simulink model "test_pi_flocking_xy_gazebo_2023a"  (R2023a)
settings: Solver=FixedStepAuto  StartTime=0.0  StopTime=inf  RelTol=1e-3
undefined symbols (not defined in the file or in its folder): angular, d_prime, DiscIntNeverNeededParam, epsilon, h, linear, R, vxobs, vyobs, vzobs, xobs, yobs, zobs
libraries: ros2lib x14, simulink x4, robotcorelib x4
(part 2 of 2)

== matlab function test_pi_flocking_xy_gazebo_2023a/Translational Control3/Flocking1/MATLAB Function4 ==
  data: xj input; yj input; zj input; vxj input; vyj input; vzj input; xk input; yk input; zk input; vxk input; vyk input; vzk input; xl input; yl input; zl input; vxl input; vyl input; vzl input; xobs parameter; yobs parameter; zobs parameter; phiBetaniknei output; R parameter; epsilon parameter; d_prime parameter; h parameter; vxobs parameter; vyobs parameter; vzobs parameter; bikve output
function [phiBetaniknei, bikve] = phiBetaFcn(xj, yj, zj, vxj, vyj, vzj, xk, yk, zk, vxk, vyk, vzk, xl, yl, zl, vxl, vyl, vzl, xobs, yobs, zobs, R, epsilon, d_prime, h, vxobs, vyobs, vzobs)
    
    dBeta = sigmaNormFun(d_prime, epsilon) ;
    
    Pj = [xj ; yj ; zj] ;
    Pk = [xk ; yk ; zk] ;
    Pl = [xl ; yl ; zl] ;
    Pc = [xobs ; yobs ; zobs] ;

    Vj = [vxj ; vyj ; vzj] ;
    Vk = [vxk ; vyk ; vzk] ;
    Vl = [vxl ; vyl ; vzl] ;
    Vc = [vxobs ; vyobs ; vzobs] ;

    % Compute closest point between the robot center and the obstacle
    % circumference (ossumming obstacles are circles)
    Pobsj = Pc + (Pj - Pc) * (R /norm(Pj - Pc)) ;
    Pobsk = Pc + (Pk - Pc) * (R /norm(Pk - Pc)) ;
    Pobsl = Pc + (Pl - Pc) * (R /norm(Pl - Pc)) ;
    %Pk = [xobs ; yobs] ;
    
    %%
    sigmaNormj = sigmaNormFun(Pobsj - Pj, epsilon) ;
    nij = gradSigmaFun(Pobsj - Pj, epsilon) ;
    
    sigmaNormk = sigmaNormFun(Pobsk - Pk, epsilon) ;
    nik = gradSigmaFun(Pobsk - Pk, epsilon) ;

    sigmaNorml = sigmaNormFun(Pobsl - Pl, epsilon) ;
    nil = gradSigmaFun(Pobsl - Pl, epsilon) ;

    %%
    sigma1j = sigma1Fun(sigmaNormj - dBeta) ;
    sigma1k = sigma1Fun(sigmaNormk - dBeta) ;
    sigma1l = sigma1Fun(sigmaNorml - dBeta) ;
            
    %%
    phiBetaj = bumpFcn(sigmaNormj/dBeta,h) * (sigma1j - 1) ;
    phiBetak = bumpFcn(sigmaNormk/dBeta,h) * (sigma1k - 1) ;
    phiBetal = bumpFcn(sigmaNorml/dBeta,h) * (sigma1l - 1) ;
            
    %% Position
    phiBetaniknei = phiBetaj.* nij + phiBetak.* nik + phiBetal.* nil;
    
    %% Velocity
    bikve = bumpFcn(sigmaNormj/dBeta,h).*(Vc + (Vj - Vc)) + bumpFcn(sigmaNormk/dBeta,h).*(Vc + (Vk - Vc)) + bumpFcn(sigmaNorml/dBeta,h).*(Vc + (Vl - Vc));
end

== matlab function test_pi_flocking_xy_gazebo_2023a/Translational Control4/Flocking1/MATLAB Function ==
  data: xi input; yi input; phiAlpha output; xj input; yj input; xk input; yk input; xl input; yl input; params input

function phiAlpha  = phiAlphaFcn(xi, yi, xj, yj, xk, yk, xl, yl, params)
    
    % Flocking parameters
    epsilon = params(1); a = params(2); b = params(3); c = params(4); d = params(5); h = params(6);

    e = abs(a - b) / sqrt(4*a*b) ;

    cAlpha = sigmaNormFun(c, epsilon) ;
    dAlpha = sigmaNormFun(d, epsilon) ;

    %%
    Pi = [xi;yi] ;
    Pj = [xj;yj] ;
    Pk = [xk;yk] ;
    Pl = [xl;yl] ;

    %%
    sigmaNormj = sigmaNormFun(Pj - Pi, epsilon) ;
    nij = gradSigmaFun(Pj - Pi, epsilon) ;
    
    sigmaNormk = sigmaNormFun(Pk - Pi, epsilon) ;
    nik = gradSigmaFun(Pk - Pi, epsilon) ;

    sigmaNorml = sigmaNormFun(Pl - Pi, epsilon) ;
    nil = gradSigmaFun(Pl - Pi, epsilon) ;

    %%
    sigma1j = sigma1Fun(sigmaNormj - dAlpha + e) ;
    sigma1k = sigma1Fun(sigmaNormk - dAlpha + e) ;
    sigma1l = sigma1Fun(sigmaNorml - dAlpha + e) ;
            
    %% Position
    phiAlphaj = 0.5 * bumpFcn(sigmaNormj/cAlpha,h) * ((a+b)*sigma1j + (a-b)) ;
    phiAlphanij = phiAlphaj.* nij ;
    
    phiAlphak = 0.5 * bumpFcn(sigmaNormk/cAlpha,h) * ((a+b)*sigma1k + (a-b)) ;
    phiAlphanik = phiAlphak.* nik ;

    phiAlphal = 0.5 * bumpFcn(sigmaNorml/cAlpha,h) * ((a+b)*sigma1l + (a-b)) ;
    phiAlphanil = phiAlphal.* nil ;

    phiAlpha = phiAlphanij + phiAlphanik + phiAlphanil;

    
end

== matlab function test_pi_flocking_xy_gazebo_2023a/Translational Control4/Flocking1/MATLAB Function1 ==
  data: phiAlpha input; phiAlpha_int input; ui_gamma input; yaw input; ieyaw input; Ui_pos output size=3; ui_yaw output; KP input; eyaw output

function [Ui_pos, ui_yaw, eyaw]  = ctrlLaw(phiAlpha, phiAlpha_int, ui_gamma, yaw, ieyaw, KP)  %, phiBetak, bikobs, phiBetanei, bikve
    
    % Control gains and parameters
    Kx = KP(1); Ky = KP(2); Kz = KP(3);
    Kix = KP(4); Kiy = KP(5); Kiz = KP(6);
    Kyaw = KP(7); Kdyaw = KP(8); Kiyaw = KP(9);
    
    hx_dot = Kx * phiAlpha(1,1) + Kix * phiAlpha_int(1,1) + ui_gamma(1,1);  %+ cBetax * (phiBetak(1,1) + phiBetanei(1,1)) + cdBetax * (bikobs(1,1) + bikve(1,1));
    hy_dot = Ky * phiAlpha(2,1) + Kiy * phiAlpha_int(2,1) + ui_gamma(2,1);  %+ cBetay * (phiBetak(2,1) + phiBetanei(2,1)) + cdBetay * (bikobs(2,1) + bikve(2,1));
    hz_dot = ui_gamma(3,1);  %+ cBetaz * (phiBetak(3,1) + phiBetanei(3,1)) + cdBetaz * (bikobs(3,1) + bikve(3,1));
    

    eyaw = 0 - yaw(1);
    deyaw = 0 - yaw(2);
    

    Ui_pos = [hx_dot; hy_dot; hz_dot] ;
    ui_yaw = Kyaw*eyaw + Kdyaw*deyaw + Kiyaw*ieyaw;

end

== matlab function test_pi_flocking_xy_gazebo_2023a/Translational Control1/Flocking1/MATLAB Function ==
  data: xi input; yi input; phiAlpha output; xj input; yj input; xk input; yk input; xl input; yl input; params input

function phiAlpha  = phiAlphaFcn(xi, yi, xj, yj, xk, yk, xl, yl, params)
    
    % Flocking parameters
    epsilon = params(1); a = params(2); b = params(3); c = params(4); d = params(5); h = params(6);

    e = abs(a - b) / sqrt(4*a*b) ;

    cAlpha = sigmaNormFun(c, epsilon) ;
    dAlpha = sigmaNormFun(d, epsilon) ;

    %%
    Pi = [xi;yi] ;
    Pj = [xj;yj] ;
    Pk = [xk;yk] ;
    Pl = [xl;yl] ;

    %%
    sigmaNormj = sigmaNormFun(Pj - Pi, epsilon) ;
    nij = gradSigmaFun(Pj - Pi, epsilon) ;
    
    sigmaNormk = sigmaNormFun(Pk - Pi, epsilon) ;
    nik = gradSigmaFun(Pk - Pi, epsilon) ;

    sigmaNorml = sigmaNormFun(Pl - Pi, epsilon) ;
    nil = gradSigmaFun(Pl - Pi, epsilon) ;

    %%
    sigma1j = sigma1Fun(sigmaNormj - dAlpha + e) ;
    sigma1k = sigma1Fun(sigmaNormk - dAlpha + e) ;
    sigma1l = sigma1Fun(sigmaNorml - dAlpha + e) ;
            
    %% Position
    phiAlphaj = 0.5 * bumpFcn(sigmaNormj/cAlpha,h) * ((a+b)*sigma1j + (a-b)) ;
    phiAlphanij = phiAlphaj.* nij ;
    
    phiAlphak = 0.5 * bumpFcn(sigmaNormk/cAlpha,h) * ((a+b)*sigma1k + (a-b)) ;
    phiAlphanik = phiAlphak.* nik ;

    phiAlphal = 0.5 * bumpFcn(sigmaNorml/cAlpha,h) * ((a+b)*sigma1l + (a-b)) ;
    phiAlphanil = phiAlphal.* nil ;

    phiAlpha = phiAlphanij + phiAlphanik + phiAlphanil;

    
end

== matlab function test_pi_flocking_xy_gazebo_2023a/Translational Control1/Flocking1/MATLAB Function1 ==
  data: phiAlpha input; phiAlpha_int input; ui_gamma input; yaw input; ieyaw input; Ui_pos output size=3; ui_yaw output; KP input; eyaw output

function [Ui_pos, ui_yaw, eyaw]  = ctrlLaw(phiAlpha, phiAlpha_int, ui_gamma, yaw, ieyaw, KP)  %, phiBetak, bikobs, phiBetanei, bikve
    
    % Control gains and parameters
    Kx = KP(1); Ky = KP(2); Kz = KP(3);
    Kix = KP(4); Kiy = KP(5); Kiz = KP(6);
    Kyaw = KP(7); Kdyaw = KP(8); Kiyaw = KP(9);
    
    hx_dot = Kx * phiAlpha(1,1) + Kix * phiAlpha_int(1,1) + ui_gamma(1,1);  %+ cBetax * (phiBetak(1,1) + phiBetanei(1,1)) + cdBetax * (bikobs(1,1) + bikve(1,1));
    hy_dot = Ky * phiAlpha(2,1) + Kiy * phiAlpha_int(2,1) + ui_gamma(2,1);  %+ cBetay * (phiBetak(2,1) + phiBetanei(2,1)) + cdBetay * (bikobs(2,1) + bikve(2,1));
    hz_dot = ui_gamma(3,1);  %+ cBetaz * (phiBetak(3,1) + phiBetanei(3,1)) + cdBetaz * (bikobs(3,1) + bikve(3,1));
    

    eyaw = 0 - yaw(1);
    deyaw = 0 - yaw(2);
    

    Ui_pos = [hx_dot; hy_dot; hz_dot] ;
    ui_yaw = Kyaw*eyaw + Kdyaw*deyaw + Kiyaw*ieyaw;

end

== matlab function test_pi_flocking_xy_gazebo_2023a/Translational Control1/Flocking1/MATLAB Function2 ==
  data: xi input; yi input; zi input; ui_gamma output; xr input; yr input; zr input; iep input size=3; ep output size=3; K_cts input

function [ui_gamma, ep] = naviFeedback(xi, yi, zi, xr, yr, zr, iep, K_cts)
    
    Kp = K_cts(1); Ki = K_cts(2);
    xmin = K_cts(3); xmax = K_cts(4);
       
    Pi = [xi ; yi ; zi] ;
    
    Pr = [xr ; yr ; zr] ;
    
    ep = Pi - Pr;
    
    ui_gamma = (-1).* satFcn(Kp.*(ep), xmin, xmax) + (-1).* satFcn(Ki.*(iep), xmin, xmax) ;
    
end

== matlab function test_pi_flocking_xy_gazebo_2023a/Translational Control1/Flocking1/MATLAB Function3 ==
  data: xi input; yi input; zi input; vxi input; vyi input; vzi input; xobs parameter; yobs parameter; zobs parameter; vxobs parameter; vyobs parameter; vzobs parameter; phiBetanik output; R parameter; epsilon parameter; d_prime parameter; h parameter; bikobs output
function [phiBetanik, bikobs] = phiBetaFcn(xi, yi, zi, vxi, vyi, vzi, xobs, yobs, zobs, vxobs, vyobs, vzobs, R, epsilon, d_prime, h)
    
    dBeta = sigmaNormFun(d_prime, epsilon) ;
    
    Pi = [xi ; yi ; zi] ;
    Pc = [xobs ; yobs ; zobs] ;
    
    Vi = [vxi ; vyi ; vzi] ;
    Vc = [vxobs ; vyobs ; vzobs] ;

    % Compute closest point between the robot center and the obstacle
    % circumference (ossumming obstacles are circles)
    Pk = Pc + (Pi - Pc) * (R /norm(Pi - Pc)) ;
    %Pk = [xobs ; yobs] ;
    
    sigmaNormk = sigmaNormFun(Pk - Pi, epsilon) ;
    nik = gradSigmaFun(Pk - Pi, epsilon) ;
    
    sigma1k = sigma1Fun(sigmaNormk - dBeta) ;
    
    %% Position
    phiBetak = bumpFcn(sigmaNormk/dBeta,h) * (sigma1k - 1) ;
    phiBetanik = phiBetak.* nik ;
    
    %% Velocity
    bikobs = bumpFcn(sigmaNormk/dBeta,h).*(Vc + (Vi - Vc));
end

== matlab function test_pi_flocking_xy_gazebo_2023a/Translational Control1/Flocking1/MATLAB Function4 ==
  data: xj input; yj input; zj input; vxj input; vyj input; vzj input; xk input; yk input; zk input; vxk input; vyk input; vzk input; xl input; yl input; zl input; vxl input; vyl input; vzl input; xobs parameter; yobs parameter; zobs parameter; phiBetaniknei output; R parameter; epsilon parameter; d_prime parameter; h parameter; vxobs parameter; vyobs parameter; vzobs parameter; bikve output
function [phiBetaniknei, bikve] = phiBetaFcn(xj, yj, zj, vxj, vyj, vzj, xk, yk, zk, vxk, vyk, vzk, xl, yl, zl, vxl, vyl, vzl, xobs, yobs, zobs, R, epsilon, d_prime, h, vxobs, vyobs, vzobs)
    
    dBeta = sigmaNormFun(d_prime, epsilon) ;
    
    Pj = [xj ; yj ; zj] ;
    Pk = [xk ; yk ; zk] ;
    Pl = [xl ; yl ; zl] ;
    Pc = [xobs ; yobs ; zobs] ;

    Vj = [vxj ; vyj ; vzj] ;
    Vk = [vxk ; vyk ; vzk] ;
    Vl = [vxl ; vyl ; vzl] ;
    Vc = [vxobs ; vyobs ; vzobs] ;

    % Compute closest point between the robot center and the obstacle
    % circumference (ossumming obstacles are circles)
    Pobsj = Pc + (Pj - Pc) * (R /norm(Pj - Pc)) ;
    Pobsk = Pc + (Pk - Pc) * (R /norm(Pk - Pc)) ;
    Pobsl = Pc + (Pl - Pc) * (R /norm(Pl - Pc)) ;
    %Pk = [xobs ; yobs] ;
    
    %%
    sigmaNormj = sigmaNormFun(Pobsj - Pj, epsilon) ;
    nij = gradSigmaFun(Pobsj - Pj, epsilon) ;
    
    sigmaNormk = sigmaNormFun(Pobsk - Pk, epsilon) ;
    nik = gradSigmaFun(Pobsk - Pk, epsilon) ;

    sigmaNorml = sigmaNormFun(Pobsl - Pl, epsilon) ;
    nil = gradSigmaFun(Pobsl - Pl, epsilon) ;

    %%
    sigma1j = sigma1Fun(sigmaNormj - dBeta) ;
    sigma1k = sigma1Fun(sigmaNormk - dBeta) ;
    sigma1l = sigma1Fun(sigmaNorml - dBeta) ;
            
    %%
    phiBetaj = bumpFcn(sigmaNormj/dBeta,h) * (sigma1j - 1) ;
    phiBetak = bumpFcn(sigmaNormk/dBeta,h) * (sigma1k - 1) ;
    phiBetal = bumpFcn(sigmaNorml/dBeta,h) * (sigma1l - 1) ;
            
    %% Position
    phiBetaniknei = phiBetaj.* nij + phiBetak.* nik + phiBetal.* nil;
    
    %% Velocity
    bikve = bumpFcn(sigmaNormj/dBeta,h).*(Vc + (Vj - Vc)) + bumpFcn(sigmaNormk/dBeta,h).*(Vc + (Vk - Vc)) + bumpFcn(sigmaNorml/dBeta,h).*(Vc + (Vl - Vc));
end

== matlab function test_pi_flocking_xy_gazebo_2023a/Translational Control4/Flocking1/MATLAB Function2 ==
  data: xi input; yi input; zi input; ui_gamma output; xr input; yr input; zr input; iep input size=3; ep output size=3; K_cts input

function [ui_gamma, ep] = naviFeedback(xi, yi, zi, xr, yr, zr, iep, K_cts)
    
    Kp = K_cts(1); Ki = K_cts(2);
    xmin = K_cts(3); xmax = K_cts(4);
       
    Pi = [xi ; yi ; zi] ;
    
    Pr = [xr ; yr ; zr] ;
    
    ep = Pi - Pr;
    
    ui_gamma = (-1).* satFcn(Kp.*(ep), xmin, xmax) + (-1).* satFcn(Ki.*(iep), xmin, xmax) ;
    
end

== matlab function test_pi_flocking_xy_gazebo_2023a/Translational Control4/Flocking1/MATLAB Function3 ==
  data: xi input; yi input; zi input; vxi input; vyi input; vzi input; xobs parameter; yobs parameter; zobs parameter; vxobs parameter; vyobs parameter; vzobs parameter; phiBetanik output; R parameter; epsilon parameter; d_prime parameter; h parameter; bikobs output
function [phiBetanik, bikobs] = phiBetaFcn(xi, yi, zi, vxi, vyi, vzi, xobs, yobs, zobs, vxobs, vyobs, vzobs, R, epsilon, d_prime, h)
    
    dBeta = sigmaNormFun(d_prime, epsilon) ;
    
    Pi = [xi ; yi ; zi] ;
    Pc = [xobs ; yobs ; zobs] ;
    
    Vi = [vxi ; vyi ; vzi] ;
    Vc = [vxobs ; vyobs ; vzobs] ;

    % Compute closest point between the robot center and the obstacle
    % circumference (ossumming obstacles are circles)
    Pk = Pc + (Pi - Pc) * (R /norm(Pi - Pc)) ;
    %Pk = [xobs ; yobs] ;
    
    sigmaNormk = sigmaNormFun(Pk - Pi, epsilon) ;
    nik = gradSigmaFun(Pk - Pi, epsilon) ;
    
    sigma1k = sigma1Fun(sigmaNormk - dBeta) ;
    
    %% Position
    phiBetak = bumpFcn(sigmaNormk/dBeta,h) * (sigma1k - 1) ;
    phiBetanik = phiBetak.* nik ;
    
    %% Velocity
    bikobs = bumpFcn(sigmaNormk/dBeta,h).*(Vc + (Vi - Vc));
end

== matlab function test_pi_flocking_xy_gazebo_2023a/Translational Control4/Flocking1/MATLAB Function4 ==
  data: xj input; yj input; zj input; vxj input; vyj input; vzj input; xk input; yk input; zk input; vxk input; vyk input; vzk input; xl input; yl input; zl input; vxl input; vyl input; vzl input; xobs parameter; yobs parameter; zobs parameter; phiBetaniknei output; R parameter; epsilon parameter; d_prime parameter; h parameter; vxobs parameter; vyobs parameter; vzobs parameter; bikve output
function [phiBetaniknei, bikve] = phiBetaFcn(xj, yj, zj, vxj, vyj, vzj, xk, yk, zk, vxk, vyk, vzk, xl, yl, zl, vxl, vyl, vzl, xobs, yobs, zobs, R, epsilon, d_prime, h, vxobs, vyobs, vzobs)
    
    dBeta = sigmaNormFun(d_prime, epsilon) ;
    
    Pj = [xj ; yj ; zj] ;
    Pk = [xk ; yk ; zk] ;
    Pl = [xl ; yl ; zl] ;
    Pc = [xobs ; yobs ; zobs] ;

    Vj = [vxj ; vyj ; vzj] ;
    Vk = [vxk ; vyk ; vzk] ;
    Vl = [vxl ; vyl ; vzl] ;
    Vc = [vxobs ; vyobs ; vzobs] ;

    % Compute closest point between the robot center and the obstacle
    % circumference (ossumming obstacles are circles)
    Pobsj = Pc + (Pj - Pc) * (R /norm(Pj - Pc)) ;
    Pobsk = Pc + (Pk - Pc) * (R /norm(Pk - Pc)) ;
    Pobsl = Pc + (Pl - Pc) * (R /norm(Pl - Pc)) ;
    %Pk = [xobs ; yobs] ;
    
    %%
    sigmaNormj = sigmaNormFun(Pobsj - Pj, epsilon) ;
    nij = gradSigmaFun(Pobsj - Pj, epsilon) ;
    
    sigmaNormk = sigmaNormFun(Pobsk - Pk, epsilon) ;
    nik = gradSigmaFun(Pobsk - Pk, epsilon) ;

    sigmaNorml = sigmaNormFun(Pobsl - Pl, epsilon) ;
    nil = gradSigmaFun(Pobsl - Pl, epsilon) ;

    %%
    sigma1j = sigma1Fun(sigmaNormj - dBeta) ;
    sigma1k = sigma1Fun(sigmaNormk - dBeta) ;
    sigma1l = sigma1Fun(sigmaNorml - dBeta) ;
            
    %%
    phiBetaj = bumpFcn(sigmaNormj/dBeta,h) * (sigma1j - 1) ;
    phiBetak = bumpFcn(sigmaNormk/dBeta,h) * (sigma1k - 1) ;
    phiBetal = bumpFcn(sigmaNorml/dBeta,h) * (sigma1l - 1) ;
            
    %% Position
    phiBetaniknei = phiBetaj.* nij + phiBetak.* nik + phiBetal.* nil;
    
    %% Velocity
    bikve = bumpFcn(sigmaNormj/dBeta,h).*(Vc + (Vj - Vc)) + bumpFcn(sigmaNormk/dBeta,h).*(Vc + (Vk - Vc)) + bumpFcn(sigmaNorml/dBeta,h).*(Vc + (Vl - Vc));
end

== matlab function test_pi_flocking_xy_gazebo_2023a/Subsystem/dist_AVT ==
  data: meas input; u_B input; dU output; dAVT output; avt_pars input
function [dU,dAVT]  = fcn(meas, u_B, avt_pars)

%Vector separation
d1 = meas(1);
d2 = meas(2);
d3 = meas(3);

avtpars = avt_pars(1:4);
inc = avtpars(1);
dec = avtpars(2);
min = avtpars(3);
max = avtpars(4);

%% memory variables
d_avt1 = u_B(1);
adjustment1 = u_B(2);
s_adjust1 = u_B(3);

d_avt2 = u_B(4);
adjustment2 = u_B(5);
s_adjust2 = u_B(6);

d_avt3 = u_B(7);
adjustment3 = u_B(8);
s_adjust3 = u_B(9);

%%
du1 = AVTfun(d_avt1, d1, adjustment1, s_adjust1, min, max, inc, dec);

du2 = AVTfun(d_avt2, d2, adjustment2, s_adjust2, min, max, inc, dec);

du3 = AVTfun(d_avt3, d3, adjustment3, s_adjust3, min, max, inc, dec);

dU = [du1;du2;du3];
dAVT = [du1(1);du2(1);du3(1)];

== matlab function test_pi_flocking_xy_gazebo_2023a/Subsystem/MATLAB Function6 ==
  data: X1 input; X2 input; X3 input; d_meas input; xyz output
function xyz = fcn(X1, X2, X3, d_meas)

%% Extract data from vectors
states1 = X1(1:3);
x1 = states1(1);
y1 = states1(2);
z1 = states1(3);

states2 = X2(1:3);
x2 = states2(1);
y2 = states2(2);
z2 = states2(3);

states3 = X3(1:3);
x3 = states3(1);
y3 = states3(2);
z3 = states3(3);

r1 = d_meas(1);
r2 = d_meas(2);
r3 = d_meas(3);

xyz = multi_fun(x1, y1, r1, x2, y2, r2, x3, y3, r3);

== matlab function test_pi_flocking_xy_gazebo_2023a/MATLAB Function1 ==
  data: sec input; gaz_time output; nanosec input
function gaz_time = fcn(sec, nanosec)

nanosec1 = double(nanosec)/1000000000; %*10^(-9);

sec1 = double(sec);

gaz_time = sec1 + nanosec1;
